simulink model "gamma_block"  (R2019a)
settings: Solver=VariableStepAuto  StartTime=0.0  StopTime=10.0  RelTol=1e-3
undefined symbols (not defined in the file): r_bPGamR, V_gamma
settings Model: Creator=rache  LastModifiedBy=rache
settings DataIOCC: ReturnWorkspaceOutputs=off
settings DebuggingCC: ArithmeticOperatorsInVariantConditions=warning

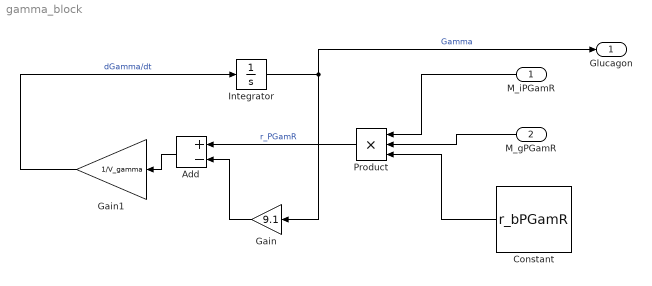
== system gamma_block ==
  M_iPGamR : Inport
  M_gPGamR : Inport  Port=2
  Add : Sum  Inputs=+-
  Constant : Constant  Value=r_bPGamR
  Gain : Gain  Gain=9.1
  Gain1 : Gain  Gain=1/V_gamma
  Integrator : Integrator
  Product : Product  Inputs=3
  Glucagon : Outport
  wires:
  Add/1 -> Gain1/1
  Constant/1 -> Product/3
  M_gPGamR/1 -> Product/2
  M_iPGamR/1 -> Product/1
  Product/1 -> Add/1  "r_PGamR"
  Integrator/1 -> Glucagon/1, Gain/1  "Gamma"
  Gain/1 -> Add/2
  Gain1/1 -> Integrator/1  "dGamma/dt"
